simulink model "coupled_tanks_sim"  (R2019a)
settings: Solver=VariableStepAuto  StartTime=0.0  StopTime=inf  RelTol=1e-3
values from neighbouring files (symbols this model uses):
  L1 = L(1)    [run_coupled_tanks.m]    (also in simulator.m = readLevels(conn,0)*6.25)
  L2 = L(2)    [run_coupled_tanks.m]    (also in simulator.m = readLevels(conn,1)*6.25)
settings Model: Creator=jeanmarioml  LastModifiedBy=jeanmarioml
settings OptimizationCC: OptimizeBlockIOStorage=off  BufferReuse=off  GlobalBufferReuse=off  ExpressionFolding=off  LocalBlockOutputs=off  OptimizeDataStoreBuffers=off  BusAssignmentInplaceUpdate=off

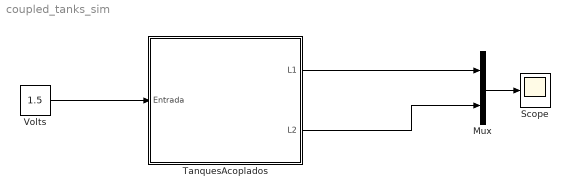
== system coupled_tanks_sim ==
  Mux : Mux  Inputs=2
  Scope : Scope
  TanquesAcoplados : Subsystem  TreatAsAtomicUnit=on  SystemSampleTime=0.01
  Volts : Constant  Value=1.5  SampleTime=0.01
  wires:
  TanquesAcoplados/2("L2 ") -> Mux/2
  Volts/1 -> TanquesAcoplados/1(Entrada)
  TanquesAcoplados/1(L1) -> Mux/1
  Mux/1 -> Scope/1

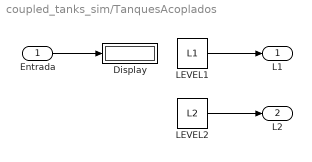
== system coupled_tanks_sim/TanquesAcoplados ==
  Entrada : Inport
  Display : Display
  LEVEL1 : Constant  Value=L1  SampleTime=0.01
  LEVEL2 : Constant  Value=L2  SampleTime=0.01
  L1 : Outport
  "L2 " : Outport  Port=2
  wires:
  LEVEL1/1 -> L1/1
  LEVEL2/1 -> "L2 "/1
  Entrada/1 -> Display/1
